simulink model "diab_for_stat__2016"  (R2016b)
settings: Solver=VariableStepAuto  StartTime=0.0  StopTime=6  RelTol=1e-6  EnableMultiTasking=on
settings Model: Creator=Alex  LastModifiedBy=alex_
settings OptimizationCC: LifeSpan=inf
settings DebuggingCC: SFUnexpectedBacktrackingDiag=warning  SFNoUnconditionalDefaultTransitionDiag=warning  SFExecutionAtInitializationDiag=none
settings GRTTargetCC: TargetLangStandard=C89/C90 (ANSI)  GeneratePreprocessorConditionals=Disable all
settings ConfigComp: CovMetricSettings=dw  CovHtmlReporting=on  CovSaveCumulativeToWorkspaceVar=on  CovSaveSingleToWorkspaceVar=on  CovExternalEMLEnable=off

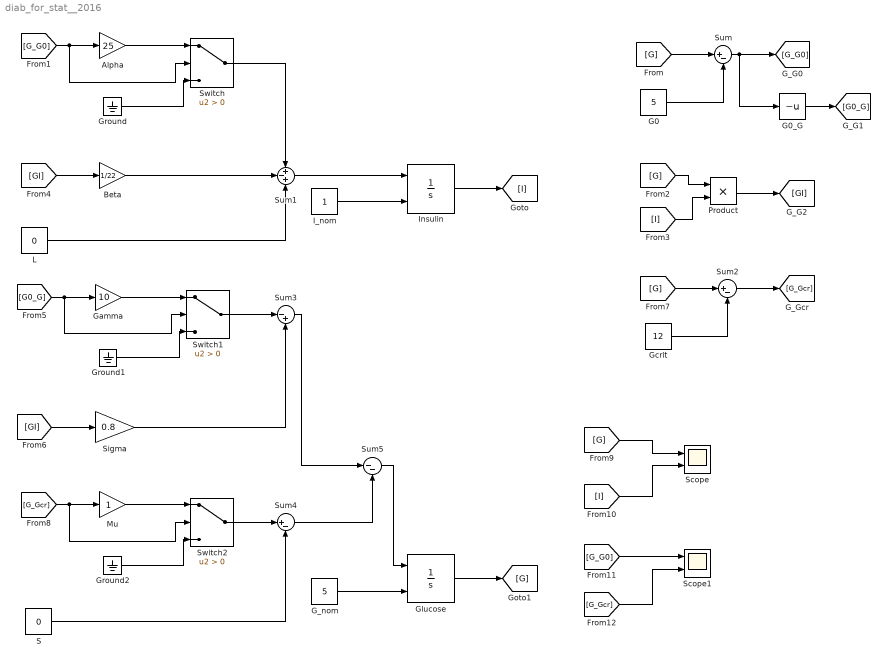
== system diab_for_stat__2016 ==
  Alpha : Gain  Gain=25
  Beta : Gain  Gain=1/22
  G0 : Constant  Value=5
  G0_G : UnaryMinus
  G_nom : Constant  Value=5
  Gamma : Gain  Gain=10
  Gcrit : Constant  Value=12
  Glucose : Integrator  InitialConditionSource=external
  Ground : Ground
  Ground1 : Ground
  Ground2 : Ground
  I_nom : Constant
  Insulin : Integrator  InitialConditionSource=external
  L : Constant  Value=0
  Mu : Gain
  Product : Product
  S : Constant  Value=0
  Scope : Scope  NumInputPorts=2
  Scope1 : Scope  NumInputPorts=2
  Sigma : Gain  Gain=0.8
  Sum : Sum  Inputs=|+-
  Sum1 : Sum  Inputs=+-+
  Sum2 : Sum  Inputs=|+-
  Sum3 : Sum  Inputs=|-+
  Sum4 : Sum  Inputs=|+-
  Sum5 : Sum  Inputs=|--
  Switch : Switch  Criteria=u2 > Threshold
  Switch1 : Switch  Criteria=u2 > Threshold
  Switch2 : Switch  Criteria=u2 > Threshold
  wires:
  I_nom/1 -> Insulin/2
  G_nom/1 -> Glucose/2
  Insulin/1 -> [I]
  Glucose/1 -> [G]
  G0/1 -> Sum/2
  [G] -> Sum/1
  Sum/1 -> G0_G/1, [G_G0]
  G0_G/1 -> [G0_G]
  [G_G0] -> Switch/2, Alpha/1
  Alpha/1 -> Switch/1
  Ground/1 -> Switch/3
  [G] -> Product/1
  [I] -> Product/2
  Product/1 -> [GI]
  [GI] -> Beta/1
  Switch/1 -> Sum1/1
  Beta/1 -> Sum1/2
  L/1 -> Sum1/3
  Sum1/1 -> Insulin/1
  [G0_G] -> Gamma/1, Switch1/2
  Gamma/1 -> Switch1/1
  Ground1/1 -> Switch1/3
  [GI] -> Sigma/1
  Gcrit/1 -> Sum2/2
  [G] -> Sum2/1
  Sum2/1 -> [G_Gcr]
  [G_Gcr] -> Switch2/2, Mu/1
  Mu/1 -> Switch2/1
  Ground2/1 -> Switch2/3
  Switch1/1 -> Sum3/1
  Sigma/1 -> Sum3/2
  Switch2/1 -> Sum4/1
  S/1 -> Sum4/2
  Sum3/1 -> Sum5/1
  Sum4/1 -> Sum5/2
  Sum5/1 -> Glucose/1
  [I] -> Scope/2
  [G] -> Scope/1
  [G_G0] -> Scope1/1
  [G_Gcr] -> Scope1/2
